simulink model "SIMULINKGRAPHS"  (R2016a)
settings: Solver=VariableStepAuto  StartTime=0.0  StopTime=200  RelTol=1e-3
values from neighbouring files (symbols this model uses):
  c = 1    [main.m]    (also in old_vehicle_suspension_model.m = 1000; plotsusp.m = 0.045; wheel_plot.m = 0.3*w4)
  k = 1000    [old_vehicle_suspension_model.m]
undefined symbols (not defined in the file or in its folder): L, m
settings Model: Creator=chris  LastModifiedBy=chris

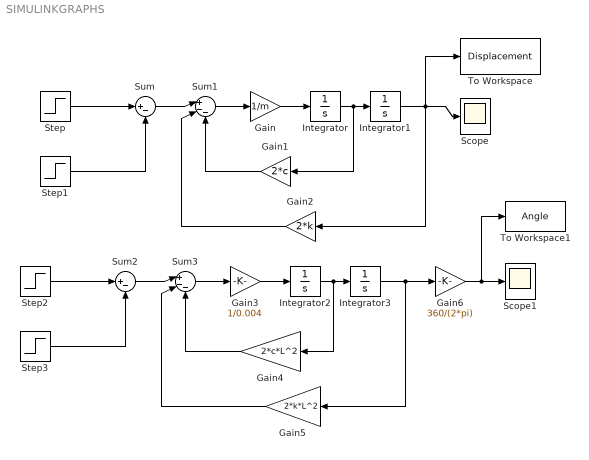
== system SIMULINKGRAPHS ==
  Gain : Gain  Gain=1/m
  Gain1 : Gain  Gain=2*c
  Gain2 : Gain  Gain=2*k
  Gain3 : Gain  Gain=1/0.004
  Gain4 : Gain  Gain=2*c*L^2
  Gain5 : Gain  Gain=2*k*L^2
  Gain6 : Gain  Gain=360/(2*pi)
  Integrator{,1..3} (4 alike) : Integrator
  Scope : Scope
  Scope1 : Scope
  Step : Step  After=0.05  SampleTime=0
  Step1 : Step  Time=20  After=0.05  SampleTime=0
  Step2 : Step  After=0.05  SampleTime=0
  Step3 : Step  Time=20  After=0.05  SampleTime=0
  Sum : Sum  Inputs=|+-
  Sum1 : Sum  Inputs=|+--
  Sum2 : Sum  Inputs=|+-
  Sum3 : Sum  Inputs=|+--
  To Workspace : ToWorkspace  VariableName=Displacement  SaveFormat=Timeseries  SampleTime=-1
      settings: Save2DSignal=2-D array (concatenate along first dimension)
  To Workspace1 : ToWorkspace  VariableName=Angle  SaveFormat=Timeseries  SampleTime=-1
      settings: Save2DSignal=2-D array (concatenate along first dimension)
  wires:
  Step/1 -> Sum/1
  Step1/1 -> Sum/2
  Sum/1 -> Sum1/1
  Sum1/1 -> Gain/1
  Gain/1 -> Integrator/1
  Integrator/1 -> Gain1/1, Integrator1/1
  Integrator1/1 -> To Workspace/1, Scope/1, Gain2/1
  Gain1/1 -> Sum1/3
  Gain2/1 -> Sum1/2
  Step2/1 -> Sum2/1
  Step3/1 -> Sum2/2
  Sum2/1 -> Sum3/1
  Sum3/1 -> Gain3/1
  Gain3/1 -> Integrator2/1
  Integrator2/1 -> Gain4/1, Integrator3/1
  Integrator3/1 -> Gain6/1, Gain5/1
  Gain4/1 -> Sum3/3
  Gain5/1 -> Sum3/2
  Gain6/1 -> To Workspace1/1, Scope1/1
